simulink model "Question_2"  (R2024b)
settings: Solver=VariableStepAuto  StartTime=0.0  StopTime=10.0  RelTol=1e-3
model workspace (MAT data in the model file):
  J_Inertia = 60
  K = 0.5
  L = 1e-06
  R = 0.3
  k = 0.5
settings Model: Creator=Sagar  LastModifiedBy=Sagar

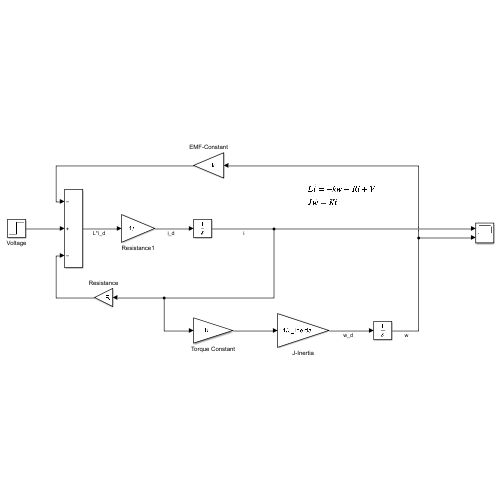
[thumbnail: Simulink's stored preview of the top-level diagram]
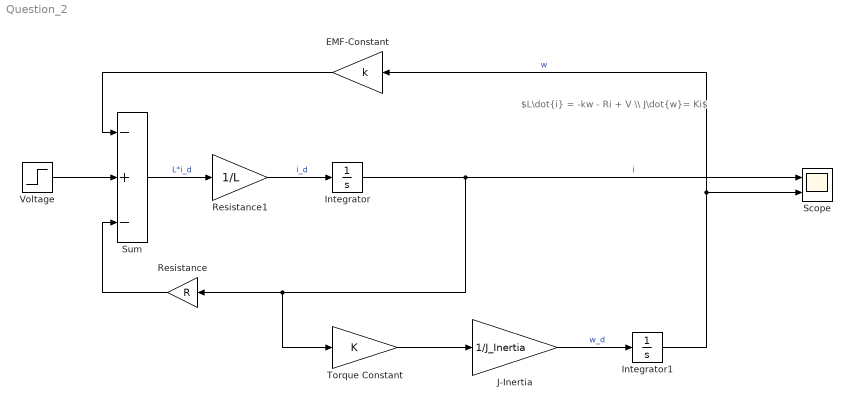
== system Question_2 ==
  note: $L\dot{i} = -kw - Ri + V \\ J\dot{w}= Ki$
  EMF-Constant : Gain  Gain=k
  Integrator : Integrator
  Integrator1 : Integrator
  J-Inertia : Gain  Gain=1/J_Inertia
  Resistance : Gain  Gain=R
  Resistance1 : Gain  Gain=1/L
  Scope : Scope  NumInputPorts=2
  Sum : Sum  Inputs=-+-
  Torque Constant : Gain  Gain=K
  Voltage : Step  SampleTime=0
  wires:
  Resistance/1 -> Sum/3
  Torque Constant/1 -> J-Inertia/1
  Integrator/1 -> Torque Constant/1, Resistance/1, Scope/1  "i"
  Integrator1/1 -> Scope/2, EMF-Constant/1  "w"
  Voltage/1 -> Sum/2
  EMF-Constant/1 -> Sum/1
  J-Inertia/1 -> Integrator1/1  "w_d"
  Resistance1/1 -> Integrator/1  "i_d"
  Sum/1 -> Resistance1/1  "L*i_d"
